simulink model "lab2part2"  (R2018a)
settings: Solver=VariableStepAuto  StartTime=0.0  StopTime=10.0  RelTol=1e-3
libraries: simulink x2
settings Model: Creator=wardzin3  LastModifiedBy=yakobovi

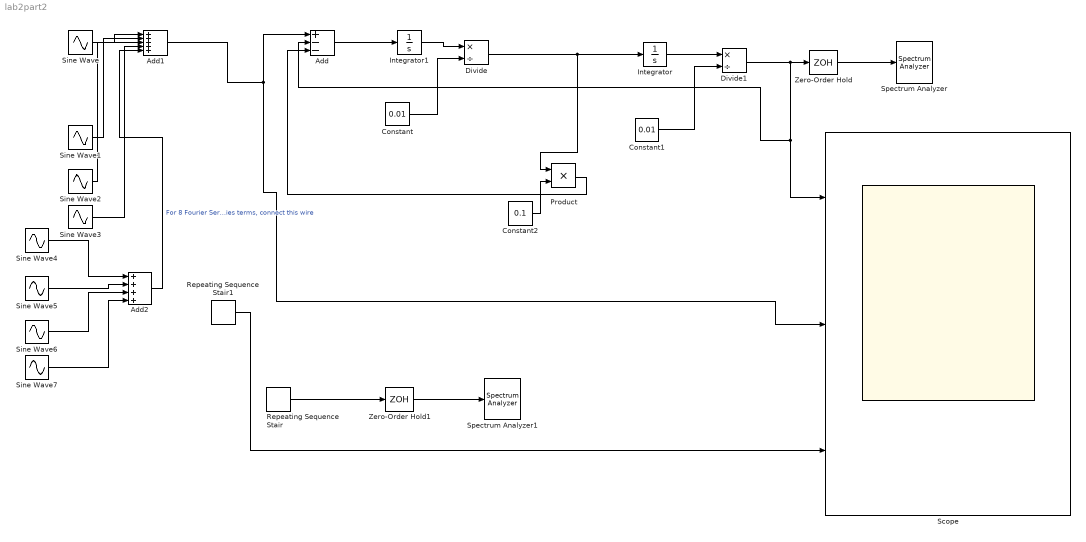
== system lab2part2 ==
  Add : Sum  Inputs=+--
  Add1 : Sum  Inputs=+++++
  Add2 : Sum  Inputs=++++
  Constant : Constant  Value=0.01
  Constant1 : Constant  Value=0.01
  Constant2 : Constant  Value=0.1
  Divide : Product  Inputs=*/
  Divide1 : Product  Inputs=*/
  Integrator : Integrator
  Integrator1 : Integrator
  Product : Product
  Repeating Sequence Stair : simulink/Sources/Repeating Sequence Stair  OutValues=[-1 1]  tsamp=1/64  OutMin=[]  OutMax=[]  OutDataTypeStr=double  OutputDataTypeScalingMode=double  OutDataType=fixdt(0,8)  ConRadixGroup=Best Precision: Vector-wise  OutScaling=2^-12
  Repeating Sequence Stair1 : simulink/Sources/Repeating Sequence Stair  OutValues=[1 -1]  tsamp=1/64  OutMin=[]  OutMax=[]  OutDataTypeStr=double  OutputDataTypeScalingMode=double  OutDataType=fixdt(0,8)  ConRadixGroup=Best Precision: Vector-wise  OutScaling=2^-12
  Scope : Scope  NumInputPorts=3
  Sine Wave : Sin  Amplitude=4/pi  Frequency=64*pi  SampleTime=2^(-14)
  Sine Wave1 : Sin  Amplitude=4/(3*pi)  Frequency=192*pi  SampleTime=2^(-14)
  Sine Wave2 : Sin  Amplitude=4/(5*pi)  Frequency=320*pi  SampleTime=2^(-14)
  Sine Wave3 : Sin  Amplitude=4/(7*pi)  Frequency=448*pi  SampleTime=2^(-14)
  Sine Wave4 : Sin  Amplitude=4/(9*pi)  Frequency=64*pi*9  SampleTime=2^(-14)
  Sine Wave5 : Sin  Amplitude=4/(11*pi)  Frequency=64*pi*11  SampleTime=2^(-14)
  Sine Wave6 : Sin  Amplitude=4/(13*pi)  Frequency=64*pi*13  SampleTime=2^(-14)
  Sine Wave7 : Sin  Amplitude=4/(15*pi)  Frequency=64*pi*15  SampleTime=2^(-14)
  Spectrum Analyzer : SpectrumAnalyzer
  Spectrum Analyzer1 : SpectrumAnalyzer
  Zero-Order Hold : ZeroOrderHold  SampleTime=2^(-10)
  Zero-Order Hold1 : ZeroOrderHold  SampleTime=2^(-10)
  wires:
  Integrator/1 -> Divide1/1
  Constant1/1 -> Divide1/2
  Constant/1 -> Divide/2
  Integrator1/1 -> Divide/1
  Add/1 -> Integrator1/1
  Divide/1 -> Product/1, Integrator/1
  Constant2/1 -> Product/2
  Divide1/1 -> Add/2, Scope/1, Zero-Order Hold/1
  Zero-Order Hold/1 -> Spectrum Analyzer/1
  Product/1 -> Add/3
  Zero-Order Hold1/1 -> Spectrum Analyzer1/1
  Repeating Sequence Stair/1 -> Zero-Order Hold1/1
  Sine Wave/1 -> Add1/1
  Sine Wave1/1 -> Add1/2
  Sine Wave2/1 -> Add1/3
  Sine Wave3/1 -> Add1/4
  Add1/1 -> Add/1, Scope/2
  Sine Wave6/1 -> Add2/3
  Sine Wave5/1 -> Add2/2
  Sine Wave7/1 -> Add2/4
  Sine Wave4/1 -> Add2/1
  Repeating Sequence Stair1/1 -> Scope/3
  Add2/1 -> Add1/5  "For 8 Fourier Series terms, connect this wire"
